simulink model "fig"  (R2019b)
settings: Solver=VariableStepAuto  StartTime=0.0  StopTime=10.0  RelTol=1e-3
values from neighbouring files (symbols this model uses):
  D = 1    [ex01.m]
  J = 1    [ex01.m]
  Kt = 1    [ex01.m]
  L = 1    [ex01.m]
  R = 1    [ex01.m]
settings Model: Creator=ryoga  LastModifiedBy=ryoga

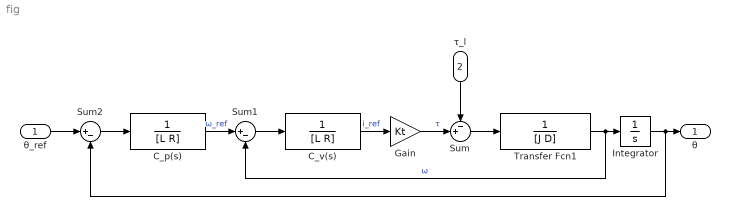
== system fig ==
  θ_ref : Inport
  τ_l : Inport  Port=2
  C_p(s) : TransferFcn  Denominator=[L R]  ContinuousStateAttributes='C_i'
  C_v(s) : TransferFcn  Denominator=[L R]  ContinuousStateAttributes='C_i'
  Gain : Gain  Gain=Kt
  Integrator : Integrator
  Sum : Sum  Inputs=-+|
  Sum1 : Sum  Inputs=|+-
  Sum2 : Sum  Inputs=|+-
  Transfer Fcn1 : TransferFcn  Denominator=[J D]
  θ : Outport
  wires:
  Sum/1 -> Transfer Fcn1/1
  C_v(s)/1 -> Gain/1  "i_ref"
  τ_l/1 -> Sum/1
  Gain/1 -> Sum/2  "τ"
  Sum1/1 -> C_v(s)/1
  θ_ref/1 -> Sum2/1
  Sum2/1 -> C_p(s)/1
  C_p(s)/1 -> Sum1/1  "ω_ref"
  Integrator/1 -> Sum2/2, θ/1
  Transfer Fcn1/1 -> Sum1/2, Integrator/1  "ω"
